simulink library "ProjectBlocks"  (R2016a)
settings: Solver=ode45  StartTime=0.0  StopTime=10.0  RelTol=1e-3
libraries: elec_lib x47, ProjectBlocks x9, SimscapeMacros x4, simulink x2, simulink_extras x1
settings Model: Creator=Peter  LastModifiedBy=Peter
settings DataIOCC: LimitDataPoints=on
settings DebuggingCC: AllowSymbolicDim=off

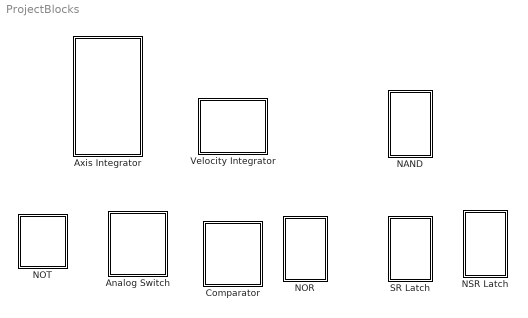
== system ProjectBlocks ==
  Analog Switch : Subsystem
  Axis Integrator : Subsystem
  Comparator : Subsystem
  NAND : Subsystem
  NOR : Subsystem
  NOT : Subsystem
  NSR Latch : Subsystem
  SR Latch : Subsystem
  Velocity Integrator : Subsystem

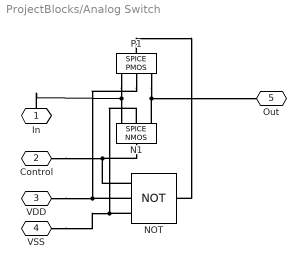
== system ProjectBlocks/Analog Switch ==
  N1 : elec_lib/Additional Components/SPICE-Compatible Components/Semiconductor Devices/SPICE NMOS  AREA=1  SCALE=1  LENGTH=7.8e-6 m  WIDTH=0.138e-3 m  AD=0.161e-8 m^2  AS=0.603e-8 m^2  PD=0 m  PS=0.478e-3 m  NRD=0.3  NRS=1  LEVEL=1  VTO=0.750 V  KP=NaN A/V^2  GAMMA=1.03 V^0.50000  PHI=0.70 V  LAMBDA=0.018 1/V  RD=NaN Ohm  RS=NaN Ohm  C_param=1  CBD=1e-18 F  CBS=1e-18 F  IS=1.206e-13 A  ND=1  PB=0.9 V  CGSO=0.94e-9 F/m  CGDO=0.59e-9 F/m  CGBO=0.138e-9 F/m  RSH=10 Ohm  CJ=0.39e-3 F/m^2  MJ=0.5  CJSW=264e-12 F/m  MJSW=0.18  JS=20e-6 A/m^2  TOX=0.055e-6 m  LD=1.6e-6 m  U0=650 cm^2/s/V  FC=0.5  NSUB=1e16 1/cm^3  TPG=1  NSS=0.7e11 1/cm^2  UEXP=0  UCRIT=1e+4 V/cm  NEFF=1  DELTA=0  VMAX=1.6e5 m/s  XJ=2.0e-6 m  NFS=1.17e11 1/cm^2  ETA=0  THETA=0 1/V  KAPPA=0.2  T_param=1  TOFFSET=0 K  TFIXED=300.15 K  TMEAS=300.15 K  IC_given=1  ICVDS=0 V  ICVGS=0 V  ICVBS=0 V  MTYPE=1
  NOT : ProjectBlocks/NOT
  P1 : elec_lib/Additional Components/SPICE-Compatible Components/Semiconductor Devices/SPICE PMOS  AREA=1  SCALE=1  LENGTH=7.8e-6 m  WIDTH=0.138e-3 m  AD=0.161e-8 m^2  AS=0.603e-8 m^2  PD=0 m  PS=0.478e-3 m  NRD=0.3  NRS=1  LEVEL=1  VTO=-0.74 V  KP=NaN A/V^2  GAMMA=0.58 V^0.50000  PHI=0.70 V  LAMBDA=.026 1/V  RD=NaN Ohm  RS=NaN Ohm  C_param=1  CBD=1e-18 F  CBS=1e-18 F  IS=1.206e-13 A  ND=1  PB=0.90 V  CGSO=0.31e-9 F/m  CGDO=0.39e-9 F/m  CGBO=0.138e-9 F/m  RSH=90 Ohm  CJ=0.18e-3 F/m^2  MJ=0.57  CJSW=322e-12 F/m  MJSW=0.33  JS=20e-6 A/m^2  TOX=0.055e-6 m  LD=0.96e-6 m  U0=260 cm^2/s/V  FC=0.5  NSUB=1e16 1/cm^3  TPG=-1  NSS=1e11 1/cm^2  UEXP=0  UCRIT=1e+4 V/cm  NEFF=1  DELTA=0  VMAX=3.0e5 m/s  XJ=1.2e-6 m  NFS=1.06e11 1/cm^2  ETA=0  THETA=0 1/V  KAPPA=0.2  T_param=1  TOFFSET=0 K  TFIXED=300.15 K  TMEAS=300.15 K  IC_given=1  ICVDS=0 V  ICVGS=0 V  ICVBS=0 V  MTYPE=-1
  In : PMIOPort  Port=1  Side=Left
  Control : PMIOPort  Port=2  Side=Left
  VDD : PMIOPort  Port=3  Side=Left
  VSS : PMIOPort  Port=4  Side=Left
  Out : PMIOPort  Port=5  Side=Right
  connections:
  P1/RConn1 -- In/RConn1 -- N1/RConn1
  N1/RConn3 -- Out/RConn1 -- P1/RConn3
  VDD/RConn1 -- NOT/LConn2 -- P1/RConn2
  VSS/RConn1 -- NOT/LConn3 -- N1/RConn2
  P1/LConn1 -- NOT/RConn1
  N1/LConn1 -- NOT/LConn1 -- Control/RConn1

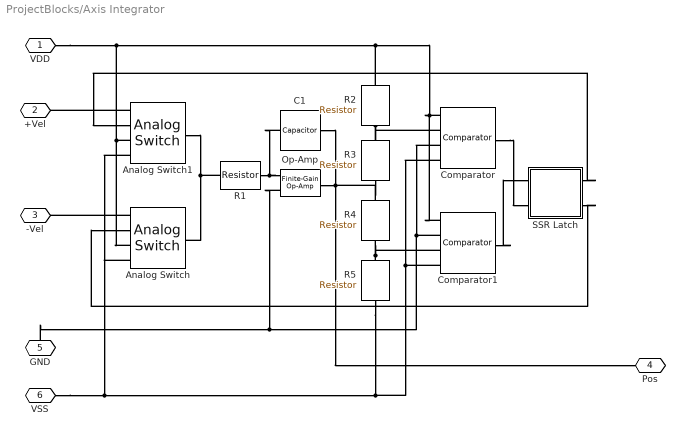
== system ProjectBlocks/Axis Integrator ==
  Analog Switch : ProjectBlocks/Analog Switch
  Analog Switch1 : ProjectBlocks/Analog Switch
  C1 : elec_lib/Passive Devices/Capacitor  enable_table=0  c=1e-6 F  Cvec=[ 1e-5 1e-6 ] F  Vvec=[ 0 10 ] V  CV_table_symmetry=1  C_tol=5  enable_C_tol=0  tol_distribution=1  nSigma=4  r=1e-6 Ohm  g=0 1/Ohm  initV=0 V  enable_operating_limits=0  operating_limit_action=2  max_working_voltage_range=[ -25 25 ] V  power_rating=1 W  enable_faults=0  fault_action=1  Cscale_faulted=100  R_faulted=0.001 Ohm  G_faulted=0 1/Ohm  tau_fault=0.001 s  enable_temporal_fault=0  t_fault=1 s  enable_behavioral_fault=0  max_permissible_voltage_range=[ -100 100 ] V  t_fail_on_voltage=1 s
  Comparator : ProjectBlocks/Comparator
  Comparator1 : ProjectBlocks/Comparator
  Op-Amp : elec_lib/Integrated Circuits/Finite-Gain Op-Amp  A=1000  Rin=1e6 Ohm  Rout=100 Ohm  Vmin=-10 V  Vmax=10 V
  R1 : elec_lib/Passive Devices/Resistor  R=100e3 Ohm  R_tol=5  enable_R_tol=0  tol_distribution=1  nSigma=4  enable_operating_limits=0  operating_limit_action=2  max_working_voltage=100 V  power_rating=1 W  enable_faults=0  fault_action=1  R_faulted=Inf Ohm  enable_temporal_fault=0  t_fault=1 s  enable_behavioral_fault=0  max_permissible_current=1 A  t_fail_on_current=1 s  noise_mode=0  sample_time=0.001 s  repeatability=1  auto_seed=736455394  user_seed=0  Tdevice=25 degC  alpha=0.00393 1/K  Tmeas=25 degC  thermal_mass=100 J/K  initial_temperature=25 degC  power_derating_T1=70 degC  power_derating_T2=155 degC  operating_temperature_range_vec=[ -50 150 ] degC
  R2 : elec_lib/Passive Devices/Resistor  R=10e3 Ohm  R_tol=5  enable_R_tol=0  tol_distribution=1  nSigma=4  enable_operating_limits=0  operating_limit_action=2  max_working_voltage=100 V  power_rating=1 W  enable_faults=0  fault_action=1  R_faulted=Inf Ohm  enable_temporal_fault=0  t_fault=1 s  enable_behavioral_fault=0  max_permissible_current=1 A  t_fail_on_current=1 s  noise_mode=0  sample_time=0.001 s  repeatability=1  auto_seed=38756620  user_seed=0  Tdevice=25 degC  alpha=0.00393 1/K  Tmeas=25 degC  thermal_mass=100 J/K  initial_temperature=25 degC  power_derating_T1=70 degC  power_derating_T2=155 degC  operating_temperature_range_vec=[ -50 150 ] degC
  R3 : elec_lib/Passive Devices/Resistor  R=5e3 Ohm  R_tol=5  enable_R_tol=0  tol_distribution=1  nSigma=4  enable_operating_limits=0  operating_limit_action=2  max_working_voltage=100 V  power_rating=1 W  enable_faults=0  fault_action=1  R_faulted=Inf Ohm  enable_temporal_fault=0  t_fault=1 s  enable_behavioral_fault=0  max_permissible_current=1 A  t_fail_on_current=1 s  noise_mode=0  sample_time=0.001 s  repeatability=1  auto_seed=726180734  user_seed=0  Tdevice=25 degC  alpha=0.00393 1/K  Tmeas=25 degC  thermal_mass=100 J/K  initial_temperature=25 degC  power_derating_T1=70 degC  power_derating_T2=155 degC  operating_temperature_range_vec=[ -50 150 ] degC
  R4 : elec_lib/Passive Devices/Resistor  R=5e3 Ohm  R_tol=5  enable_R_tol=0  tol_distribution=1  nSigma=4  enable_operating_limits=0  operating_limit_action=2  max_working_voltage=100 V  power_rating=1 W  enable_faults=0  fault_action=1  R_faulted=Inf Ohm  enable_temporal_fault=0  t_fault=1 s  enable_behavioral_fault=0  max_permissible_current=1 A  t_fail_on_current=1 s  noise_mode=0  sample_time=0.001 s  repeatability=1  auto_seed=886428727  user_seed=0  Tdevice=25 degC  alpha=0.00393 1/K  Tmeas=25 degC  thermal_mass=100 J/K  initial_temperature=25 degC  power_derating_T1=70 degC  power_derating_T2=155 degC  operating_temperature_range_vec=[ -50 150 ] degC
  R5 : elec_lib/Passive Devices/Resistor  R=10e3 Ohm  R_tol=5  enable_R_tol=0  tol_distribution=1  nSigma=4  enable_operating_limits=0  operating_limit_action=2  max_working_voltage=100 V  power_rating=1 W  enable_faults=0  fault_action=1  R_faulted=Inf Ohm  enable_temporal_fault=0  t_fault=1 s  enable_behavioral_fault=0  max_permissible_current=1 A  t_fail_on_current=1 s  noise_mode=0  sample_time=0.001 s  repeatability=1  auto_seed=3872437814  user_seed=0  Tdevice=25 degC  alpha=0.00393 1/K  Tmeas=25 degC  thermal_mass=100 J/K  initial_temperature=25 degC  power_derating_T1=70 degC  power_derating_T2=155 degC  operating_temperature_range_vec=[ -50 150 ] degC
  SSR Latch : Subsystem
  VDD : PMIOPort  Port=1  Side=Left
  +Vel : PMIOPort  Port=2  Side=Left
  -Vel : PMIOPort  Port=3  Side=Left
  Pos : PMIOPort  Port=4  Side=Right
  GND : PMIOPort  Port=5  Side=Left
  VSS : PMIOPort  Port=6  Side=Left
  connections:
  R1/RConn1 -- Op-Amp/LConn2 -- C1/RConn1
  Comparator/LConn4 -- Comparator1/LConn4 -- R5/RConn1 -- Analog Switch/LConn4 -- Analog Switch1/LConn4 -- VSS/RConn1
  Analog Switch/LConn3 -- Analog Switch1/LConn3 -- R2/LConn1 -- Comparator/LConn1 -- Comparator1/LConn1 -- VDD/RConn1
  R3/LConn1 -- R2/RConn1 -- Comparator/LConn2
  Op-Amp/LConn1 -- Comparator/LConn3 -- Comparator1/LConn2 -- GND/RConn1
  Analog Switch/LConn1 -- -Vel/RConn1
  Analog Switch1/LConn1 -- +Vel/RConn1
  R4/RConn1 -- R5/LConn1 -- Comparator1/LConn3
  R1/LConn1 -- Analog Switch1/RConn1 -- Analog Switch/RConn1
  C1/LConn1 -- R3/RConn1 -- R4/LConn1 -- Op-Amp/RConn1 -- Pos/RConn1
  SSR Latch/RConn2 -- Analog Switch/LConn2
  SSR Latch/RConn1 -- Analog Switch1/LConn2
  Comparator/RConn1 -- SSR Latch/LConn2
  Comparator1/RConn1 -- SSR Latch/LConn1

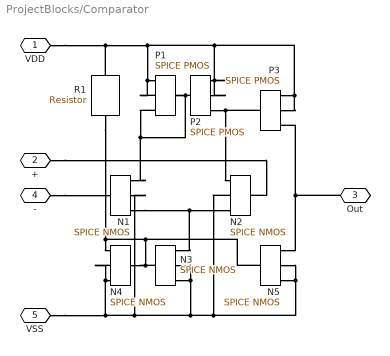
== system ProjectBlocks/Comparator ==
  N{1..5} (5 alike) : elec_lib/Additional Components/SPICE-Compatible Components/Semiconductor Devices/SPICE NMOS  AREA=1  SCALE=1  LENGTH=7.8e-6 m  WIDTH=0.138e-3 m  AD=0.161e-8 m^2  AS=0.603e-8 m^2  PD=0 m  PS=0.478e-3 m  NRD=0.3  NRS=1  LEVEL=1  VTO=0.750 V  KP=NaN A/V^2  GAMMA=1.03 V^0.50000  PHI=0.70 V  LAMBDA=0.018 1/V  RD=NaN Ohm  RS=NaN Ohm  C_param=1  CBD=1e-18 F  CBS=1e-18 F  IS=1.206e-13 A  ND=1  PB=0.9 V  CGSO=0.94e-9 F/m  CGDO=0.59e-9 F/m  CGBO=0.138e-9 F/m  RSH=10 Ohm  CJ=0.39e-3 F/m^2  MJ=0.5  CJSW=264e-12 F/m  MJSW=0.18  JS=20e-6 A/m^2  TOX=0.055e-6 m  LD=1.6e-6 m  U0=650 cm^2/s/V  FC=0.5  NSUB=1e16 1/cm^3  TPG=1  NSS=0.7e11 1/cm^2  UEXP=0  UCRIT=1e+4 V/cm  NEFF=1  DELTA=0  VMAX=1.6e5 m/s  XJ=2.0e-6 m  NFS=1.17e11 1/cm^2  ETA=0  THETA=0 1/V  KAPPA=0.2  T_param=1  TOFFSET=0 K  TFIXED=300.15 K  TMEAS=300.15 K  IC_given=1  ICVDS=0 V  ICVGS=0 V  ICVBS=0 V  MTYPE=1
  P1 : elec_lib/Additional Components/SPICE-Compatible Components/Semiconductor Devices/SPICE PMOS  AREA=1  SCALE=1  LENGTH=7.8e-6 m  WIDTH=0.138e-3 m  AD=0.161e-8 m^2  AS=0.603e-8 m^2  PD=0 m  PS=0.478e-3 m  NRD=0.3  NRS=1  LEVEL=1  VTO=-0.74 V  KP=NaN A/V^2  GAMMA=0.58 V^0.50000  PHI=0.70 V  LAMBDA=.026 1/V  RD=NaN Ohm  RS=NaN Ohm  C_param=1  CBD=1e-18 F  CBS=1e-18 F  IS=1.206e-13 A  ND=1  PB=0.90 V  CGSO=0.31e-9 F/m  CGDO=0.39e-9 F/m  CGBO=0.138e-9 F/m  RSH=90 Ohm  CJ=0.18e-3 F/m^2  MJ=0.57  CJSW=322e-12 F/m  MJSW=0.33  JS=20e-6 A/m^2  TOX=0.055e-6 m  LD=0.96e-6 m  U0=260 cm^2/s/V  FC=0.5  NSUB=1e16 1/cm^3  TPG=-1  NSS=1e11 1/cm^2  UEXP=0  UCRIT=1e+4 V/cm  NEFF=1  DELTA=0  VMAX=3.0e5 m/s  XJ=1.2e-6 m  NFS=1.06e11 1/cm^2  ETA=0  THETA=0 1/V  KAPPA=0.2  T_param=1  TOFFSET=0 K  TFIXED=300.15 K  TMEAS=300.15 K  IC_given=1  ICVDS=0 V  ICVGS=0 V  ICVBS=0 V  MTYPE=-1
  P2 : elec_lib/Additional Components/SPICE-Compatible Components/Semiconductor Devices/SPICE PMOS  AREA=1  SCALE=1  LENGTH=7.8e-6 m  WIDTH=0.138e-3 m  AD=0.161e-8 m^2  AS=0.603e-8 m^2  PD=0 m  PS=0.478e-3 m  NRD=0.3  NRS=1  LEVEL=1  VTO=-0.74 V  KP=NaN A/V^2  GAMMA=0.58 V^0.50000  PHI=0.70 V  LAMBDA=.026 1/V  RD=NaN Ohm  RS=NaN Ohm  C_param=1  CBD=1e-18 F  CBS=1e-18 F  IS=1.206e-13 A  ND=1  PB=0.90 V  CGSO=0.31e-9 F/m  CGDO=0.39e-9 F/m  CGBO=0.138e-9 F/m  RSH=90 Ohm  CJ=0.18e-3 F/m^2  MJ=0.57  CJSW=322e-12 F/m  MJSW=0.33  JS=20e-6 A/m^2  TOX=0.055e-6 m  LD=0.96e-6 m  U0=260 cm^2/s/V  FC=0.5  NSUB=1e16 1/cm^3  TPG=-1  NSS=1e11 1/cm^2  UEXP=0  UCRIT=1e+4 V/cm  NEFF=1  DELTA=0  VMAX=3.0e5 m/s  XJ=1.2e-6 m  NFS=1.06e11 1/cm^2  ETA=0  THETA=0 1/V  KAPPA=0.2  T_param=1  TOFFSET=0 K  TFIXED=300.15 K  TMEAS=300.15 K  IC_given=1  ICVDS=0 V  ICVGS=0 V  ICVBS=0 V  MTYPE=-1
  P3 : elec_lib/Additional Components/SPICE-Compatible Components/Semiconductor Devices/SPICE PMOS  AREA=1  SCALE=1  LENGTH=7.8e-6 m  WIDTH=0.138e-3 m  AD=0.161e-8 m^2  AS=0.603e-8 m^2  PD=0 m  PS=0.478e-3 m  NRD=0.3  NRS=1  LEVEL=1  VTO=-0.74 V  KP=NaN A/V^2  GAMMA=0.58 V^0.50000  PHI=0.70 V  LAMBDA=.026 1/V  RD=NaN Ohm  RS=NaN Ohm  C_param=1  CBD=1e-18 F  CBS=1e-18 F  IS=1.206e-13 A  ND=1  PB=0.90 V  CGSO=0.31e-9 F/m  CGDO=0.39e-9 F/m  CGBO=0.138e-9 F/m  RSH=90 Ohm  CJ=0.18e-3 F/m^2  MJ=0.57  CJSW=322e-12 F/m  MJSW=0.33  JS=20e-6 A/m^2  TOX=0.055e-6 m  LD=0.96e-6 m  U0=260 cm^2/s/V  FC=0.5  NSUB=1e16 1/cm^3  TPG=-1  NSS=1e11 1/cm^2  UEXP=0  UCRIT=1e+4 V/cm  NEFF=1  DELTA=0  VMAX=3.0e5 m/s  XJ=1.2e-6 m  NFS=1.06e11 1/cm^2  ETA=0  THETA=0 1/V  KAPPA=0.2  T_param=1  TOFFSET=0 K  TFIXED=300.15 K  TMEAS=300.15 K  IC_given=1  ICVDS=0 V  ICVGS=0 V  ICVBS=0 V  MTYPE=-1
  R1 : elec_lib/Passive Devices/Resistor  R=72e3 Ohm  R_tol=5  enable_R_tol=0  tol_distribution=1  nSigma=4  enable_operating_limits=0  operating_limit_action=2  max_working_voltage=100 V  power_rating=1 W  enable_faults=0  fault_action=1  R_faulted=Inf Ohm  enable_temporal_fault=0  t_fault=1 s  enable_behavioral_fault=0  max_permissible_current=1 A  t_fail_on_current=1 s  noise_mode=0  sample_time=0.001 s  repeatability=1  auto_seed=1225241502  user_seed=0  Tdevice=25 degC  alpha=0.00393 1/K  Tmeas=25 degC  thermal_mass=100 J/K  initial_temperature=25 degC  power_derating_T1=70 degC  power_derating_T2=155 degC  operating_temperature_range_vec=[ -50 150 ] degC
  VDD : PMIOPort  Port=1  Side=Left
  + : PMIOPort  Port=2  Side=Left
  Out : PMIOPort  Port=3  Side=Right
  - : PMIOPort  Port=4  Side=Left
  VSS : PMIOPort  Port=5  Side=Left
  connections:
  VSS/RConn1 -- N2/RConn2 -- N5/RConn2 -- N5/RConn1 -- N3/RConn2 -- N3/RConn1 -- N1/RConn2 -- N4/RConn2 -- N4/RConn1
  R1/RConn1 -- N3/LConn1 -- N4/LConn1 -- N5/LConn1 -- N4/RConn3
  N5/RConn3 -- Out/RConn1 -- P3/RConn3
  P2/RConn3 -- P3/LConn1 -- N2/RConn3
  +/RConn1 -- N2/LConn1
  -/RConn1 -- N1/LConn1
  P1/RConn3 -- N1/RConn3 -- P2/LConn1 -- P1/LConn1
  P2/RConn1 -- P3/RConn2 -- P3/RConn1 -- VDD/RConn1 -- R1/LConn1 -- P1/RConn2 -- P1/RConn1 -- P2/RConn2
  N1/RConn1 -- N3/RConn3 -- N2/RConn1

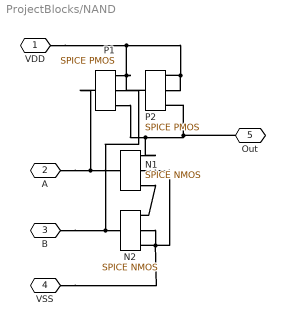
== system ProjectBlocks/NAND ==
  N1 : elec_lib/Additional Components/SPICE-Compatible Components/Semiconductor Devices/SPICE NMOS  AREA=1  SCALE=1  LENGTH=7.8e-6 m  WIDTH=0.138e-3 m  AD=0.161e-8 m^2  AS=0.603e-8 m^2  PD=0 m  PS=0.478e-3 m  NRD=0.3  NRS=1  LEVEL=1  VTO=0.750 V  KP=NaN A/V^2  GAMMA=1.03 V^0.50000  PHI=0.70 V  LAMBDA=0.018 1/V  RD=NaN Ohm  RS=NaN Ohm  C_param=1  CBD=1e-18 F  CBS=1e-18 F  IS=1.206e-13 A  ND=1  PB=0.9 V  CGSO=0.94e-9 F/m  CGDO=0.59e-9 F/m  CGBO=0.138e-9 F/m  RSH=10 Ohm  CJ=0.39e-3 F/m^2  MJ=0.5  CJSW=264e-12 F/m  MJSW=0.18  JS=20e-6 A/m^2  TOX=0.055e-6 m  LD=1.6e-6 m  U0=650 cm^2/s/V  FC=0.5  NSUB=1e16 1/cm^3  TPG=1  NSS=0.7e11 1/cm^2  UEXP=0  UCRIT=1e+4 V/cm  NEFF=1  DELTA=0  VMAX=1.6e5 m/s  XJ=2.0e-6 m  NFS=1.17e11 1/cm^2  ETA=0  THETA=0 1/V  KAPPA=0.2  T_param=1  TOFFSET=0 K  TFIXED=300.15 K  TMEAS=300.15 K  IC_given=1  ICVDS=0 V  ICVGS=0 V  ICVBS=0 V  MTYPE=1
  N2 : elec_lib/Additional Components/SPICE-Compatible Components/Semiconductor Devices/SPICE NMOS  AREA=1  SCALE=1  LENGTH=7.8e-6 m  WIDTH=0.138e-3 m  AD=0.161e-8 m^2  AS=0.603e-8 m^2  PD=0 m  PS=0.478e-3 m  NRD=0.3  NRS=1  LEVEL=1  VTO=0.750 V  KP=NaN A/V^2  GAMMA=1.03 V^0.50000  PHI=0.70 V  LAMBDA=0.018 1/V  RD=NaN Ohm  RS=NaN Ohm  C_param=1  CBD=1e-18 F  CBS=1e-18 F  IS=1.206e-13 A  ND=1  PB=0.9 V  CGSO=0.94e-9 F/m  CGDO=0.59e-9 F/m  CGBO=0.138e-9 F/m  RSH=10 Ohm  CJ=0.39e-3 F/m^2  MJ=0.5  CJSW=264e-12 F/m  MJSW=0.18  JS=20e-6 A/m^2  TOX=0.055e-6 m  LD=1.6e-6 m  U0=650 cm^2/s/V  FC=0.5  NSUB=1e16 1/cm^3  TPG=1  NSS=0.7e11 1/cm^2  UEXP=0  UCRIT=1e+4 V/cm  NEFF=1  DELTA=0  VMAX=1.6e5 m/s  XJ=2.0e-6 m  NFS=1.17e11 1/cm^2  ETA=0  THETA=0 1/V  KAPPA=0.2  T_param=1  TOFFSET=0 K  TFIXED=300.15 K  TMEAS=300.15 K  IC_given=1  ICVDS=0 V  ICVGS=0 V  ICVBS=0 V  MTYPE=1
  P1 : elec_lib/Additional Components/SPICE-Compatible Components/Semiconductor Devices/SPICE PMOS  AREA=1  SCALE=1  LENGTH=7.8e-6 m  WIDTH=0.138e-3 m  AD=0.161e-8 m^2  AS=0.603e-8 m^2  PD=0 m  PS=0.478e-3 m  NRD=0.3  NRS=1  LEVEL=1  VTO=-0.74 V  KP=NaN A/V^2  GAMMA=0.58 V^0.50000  PHI=0.70 V  LAMBDA=.026 1/V  RD=NaN Ohm  RS=NaN Ohm  C_param=1  CBD=1e-18 F  CBS=1e-18 F  IS=1.206e-13 A  ND=1  PB=0.90 V  CGSO=0.31e-9 F/m  CGDO=0.39e-9 F/m  CGBO=0.138e-9 F/m  RSH=90 Ohm  CJ=0.18e-3 F/m^2  MJ=0.57  CJSW=322e-12 F/m  MJSW=0.33  JS=20e-6 A/m^2  TOX=0.055e-6 m  LD=0.96e-6 m  U0=260 cm^2/s/V  FC=0.5  NSUB=1e16 1/cm^3  TPG=-1  NSS=1e11 1/cm^2  UEXP=0  UCRIT=1e+4 V/cm  NEFF=1  DELTA=0  VMAX=3.0e5 m/s  XJ=1.2e-6 m  NFS=1.06e11 1/cm^2  ETA=0  THETA=0 1/V  KAPPA=0.2  T_param=1  TOFFSET=0 K  TFIXED=300.15 K  TMEAS=300.15 K  IC_given=1  ICVDS=0 V  ICVGS=0 V  ICVBS=0 V  MTYPE=-1
  P2 : elec_lib/Additional Components/SPICE-Compatible Components/Semiconductor Devices/SPICE PMOS  AREA=1  SCALE=1  LENGTH=7.8e-6 m  WIDTH=0.138e-3 m  AD=0.161e-8 m^2  AS=0.603e-8 m^2  PD=0 m  PS=0.478e-3 m  NRD=0.3  NRS=1  LEVEL=1  VTO=-0.74 V  KP=NaN A/V^2  GAMMA=0.58 V^0.50000  PHI=0.70 V  LAMBDA=.026 1/V  RD=NaN Ohm  RS=NaN Ohm  C_param=1  CBD=1e-18 F  CBS=1e-18 F  IS=1.206e-13 A  ND=1  PB=0.90 V  CGSO=0.31e-9 F/m  CGDO=0.39e-9 F/m  CGBO=0.138e-9 F/m  RSH=90 Ohm  CJ=0.18e-3 F/m^2  MJ=0.57  CJSW=322e-12 F/m  MJSW=0.33  JS=20e-6 A/m^2  TOX=0.055e-6 m  LD=0.96e-6 m  U0=260 cm^2/s/V  FC=0.5  NSUB=1e16 1/cm^3  TPG=-1  NSS=1e11 1/cm^2  UEXP=0  UCRIT=1e+4 V/cm  NEFF=1  DELTA=0  VMAX=3.0e5 m/s  XJ=1.2e-6 m  NFS=1.06e11 1/cm^2  ETA=0  THETA=0 1/V  KAPPA=0.2  T_param=1  TOFFSET=0 K  TFIXED=300.15 K  TMEAS=300.15 K  IC_given=1  ICVDS=0 V  ICVGS=0 V  ICVBS=0 V  MTYPE=-1
  VDD : PMIOPort  Port=1  Side=Left
  A : PMIOPort  Port=2  Side=Left
  B : PMIOPort  Port=3  Side=Left
  VSS : PMIOPort  Port=4  Side=Left
  Out : PMIOPort  Port=5  Side=Right
  connections:
  VDD/RConn1 -- P1/RConn2 -- P1/RConn1 -- P2/RConn2 -- P2/RConn1
  N2/LConn1 -- B/RConn1 -- P2/LConn1
  N1/RConn1 -- N2/RConn3
  N2/RConn1 -- VSS/RConn1 -- N1/RConn2 -- N2/RConn2
  P1/RConn3 -- N1/RConn3 -- Out/RConn1 -- P2/RConn3
  N1/LConn1 -- A/RConn1 -- P1/LConn1

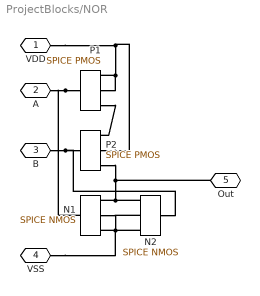
== system ProjectBlocks/NOR ==
  N1 : elec_lib/Additional Components/SPICE-Compatible Components/Semiconductor Devices/SPICE NMOS  AREA=1  SCALE=1  LENGTH=7.8e-6 m  WIDTH=0.138e-3 m  AD=0.161e-8 m^2  AS=0.603e-8 m^2  PD=0 m  PS=0.478e-3 m  NRD=0.3  NRS=1  LEVEL=1  VTO=0.750 V  KP=NaN A/V^2  GAMMA=1.03 V^0.50000  PHI=0.70 V  LAMBDA=0.018 1/V  RD=NaN Ohm  RS=NaN Ohm  C_param=1  CBD=1e-18 F  CBS=1e-18 F  IS=1.206e-13 A  ND=1  PB=0.9 V  CGSO=0.94e-9 F/m  CGDO=0.59e-9 F/m  CGBO=0.138e-9 F/m  RSH=10 Ohm  CJ=0.39e-3 F/m^2  MJ=0.5  CJSW=264e-12 F/m  MJSW=0.18  JS=20e-6 A/m^2  TOX=0.055e-6 m  LD=1.6e-6 m  U0=650 cm^2/s/V  FC=0.5  NSUB=1e16 1/cm^3  TPG=1  NSS=0.7e11 1/cm^2  UEXP=0  UCRIT=1e+4 V/cm  NEFF=1  DELTA=0  VMAX=1.6e5 m/s  XJ=2.0e-6 m  NFS=1.17e11 1/cm^2  ETA=0  THETA=0 1/V  KAPPA=0.2  T_param=1  TOFFSET=0 K  TFIXED=300.15 K  TMEAS=300.15 K  IC_given=1  ICVDS=0 V  ICVGS=0 V  ICVBS=0 V  MTYPE=1
  N2 : elec_lib/Additional Components/SPICE-Compatible Components/Semiconductor Devices/SPICE NMOS  AREA=1  SCALE=1  LENGTH=7.8e-6 m  WIDTH=0.138e-3 m  AD=0.161e-8 m^2  AS=0.603e-8 m^2  PD=0 m  PS=0.478e-3 m  NRD=0.3  NRS=1  LEVEL=1  VTO=0.750 V  KP=NaN A/V^2  GAMMA=1.03 V^0.50000  PHI=0.70 V  LAMBDA=0.018 1/V  RD=NaN Ohm  RS=NaN Ohm  C_param=1  CBD=1e-18 F  CBS=1e-18 F  IS=1.206e-13 A  ND=1  PB=0.9 V  CGSO=0.94e-9 F/m  CGDO=0.59e-9 F/m  CGBO=0.138e-9 F/m  RSH=10 Ohm  CJ=0.39e-3 F/m^2  MJ=0.5  CJSW=264e-12 F/m  MJSW=0.18  JS=20e-6 A/m^2  TOX=0.055e-6 m  LD=1.6e-6 m  U0=650 cm^2/s/V  FC=0.5  NSUB=1e16 1/cm^3  TPG=1  NSS=0.7e11 1/cm^2  UEXP=0  UCRIT=1e+4 V/cm  NEFF=1  DELTA=0  VMAX=1.6e5 m/s  XJ=2.0e-6 m  NFS=1.17e11 1/cm^2  ETA=0  THETA=0 1/V  KAPPA=0.2  T_param=1  TOFFSET=0 K  TFIXED=300.15 K  TMEAS=300.15 K  IC_given=1  ICVDS=0 V  ICVGS=0 V  ICVBS=0 V  MTYPE=1
  P1 : elec_lib/Additional Components/SPICE-Compatible Components/Semiconductor Devices/SPICE PMOS  AREA=1  SCALE=1  LENGTH=7.8e-6 m  WIDTH=0.138e-3 m  AD=0.161e-8 m^2  AS=0.603e-8 m^2  PD=0 m  PS=0.478e-3 m  NRD=0.3  NRS=1  LEVEL=1  VTO=-0.74 V  KP=NaN A/V^2  GAMMA=0.58 V^0.50000  PHI=0.70 V  LAMBDA=.026 1/V  RD=NaN Ohm  RS=NaN Ohm  C_param=1  CBD=1e-18 F  CBS=1e-18 F  IS=1.206e-13 A  ND=1  PB=0.90 V  CGSO=0.31e-9 F/m  CGDO=0.39e-9 F/m  CGBO=0.138e-9 F/m  RSH=90 Ohm  CJ=0.18e-3 F/m^2  MJ=0.57  CJSW=322e-12 F/m  MJSW=0.33  JS=20e-6 A/m^2  TOX=0.055e-6 m  LD=0.96e-6 m  U0=260 cm^2/s/V  FC=0.5  NSUB=1e16 1/cm^3  TPG=-1  NSS=1e11 1/cm^2  UEXP=0  UCRIT=1e+4 V/cm  NEFF=1  DELTA=0  VMAX=3.0e5 m/s  XJ=1.2e-6 m  NFS=1.06e11 1/cm^2  ETA=0  THETA=0 1/V  KAPPA=0.2  T_param=1  TOFFSET=0 K  TFIXED=300.15 K  TMEAS=300.15 K  IC_given=1  ICVDS=0 V  ICVGS=0 V  ICVBS=0 V  MTYPE=-1
  P2 : elec_lib/Additional Components/SPICE-Compatible Components/Semiconductor Devices/SPICE PMOS  AREA=1  SCALE=1  LENGTH=7.8e-6 m  WIDTH=0.138e-3 m  AD=0.161e-8 m^2  AS=0.603e-8 m^2  PD=0 m  PS=0.478e-3 m  NRD=0.3  NRS=1  LEVEL=1  VTO=-0.74 V  KP=NaN A/V^2  GAMMA=0.58 V^0.50000  PHI=0.70 V  LAMBDA=.026 1/V  RD=NaN Ohm  RS=NaN Ohm  C_param=1  CBD=1e-18 F  CBS=1e-18 F  IS=1.206e-13 A  ND=1  PB=0.90 V  CGSO=0.31e-9 F/m  CGDO=0.39e-9 F/m  CGBO=0.138e-9 F/m  RSH=90 Ohm  CJ=0.18e-3 F/m^2  MJ=0.57  CJSW=322e-12 F/m  MJSW=0.33  JS=20e-6 A/m^2  TOX=0.055e-6 m  LD=0.96e-6 m  U0=260 cm^2/s/V  FC=0.5  NSUB=1e16 1/cm^3  TPG=-1  NSS=1e11 1/cm^2  UEXP=0  UCRIT=1e+4 V/cm  NEFF=1  DELTA=0  VMAX=3.0e5 m/s  XJ=1.2e-6 m  NFS=1.06e11 1/cm^2  ETA=0  THETA=0 1/V  KAPPA=0.2  T_param=1  TOFFSET=0 K  TFIXED=300.15 K  TMEAS=300.15 K  IC_given=1  ICVDS=0 V  ICVGS=0 V  ICVBS=0 V  MTYPE=-1
  VDD : PMIOPort  Port=1  Side=Left
  A : PMIOPort  Port=2  Side=Left
  B : PMIOPort  Port=3  Side=Left
  VSS : PMIOPort  Port=4  Side=Left
  Out : PMIOPort  Port=5  Side=Right
  connections:
  P1/RConn3 -- P2/RConn1
  P2/RConn3 -- Out/RConn1 -- N2/RConn3 -- N1/RConn3
  B/RConn1 -- N2/LConn1 -- P2/LConn1
  A/RConn1 -- N1/LConn1 -- P1/LConn1
  VDD/RConn1 -- P2/RConn2 -- P1/RConn2 -- P1/RConn1
  VSS/RConn1 -- N2/RConn2 -- N1/RConn2 -- N2/RConn1 -- N1/RConn1

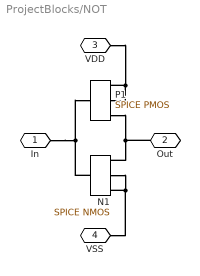
== system ProjectBlocks/NOT ==
  N1 : elec_lib/Additional Components/SPICE-Compatible Components/Semiconductor Devices/SPICE NMOS  AREA=1  SCALE=1  LENGTH=7.8e-6 m  WIDTH=0.138e-3 m  AD=0.161e-8 m^2  AS=0.603e-8 m^2  PD=0 m  PS=0.478e-3 m  NRD=0.3  NRS=1  LEVEL=1  VTO=0.750 V  KP=NaN A/V^2  GAMMA=1.03 V^0.50000  PHI=0.70 V  LAMBDA=0.018 1/V  RD=NaN Ohm  RS=NaN Ohm  C_param=1  CBD=1e-18 F  CBS=1e-18 F  IS=1.206e-13 A  ND=1  PB=0.9 V  CGSO=0.94e-9 F/m  CGDO=0.59e-9 F/m  CGBO=0.138e-9 F/m  RSH=10 Ohm  CJ=0.39e-3 F/m^2  MJ=0.5  CJSW=264e-12 F/m  MJSW=0.18  JS=20e-6 A/m^2  TOX=0.055e-6 m  LD=1.6e-6 m  U0=650 cm^2/s/V  FC=0.5  NSUB=1e16 1/cm^3  TPG=1  NSS=0.7e11 1/cm^2  UEXP=0  UCRIT=1e+4 V/cm  NEFF=1  DELTA=0  VMAX=1.6e5 m/s  XJ=2.0e-6 m  NFS=1.17e11 1/cm^2  ETA=0  THETA=0 1/V  KAPPA=0.2  T_param=1  TOFFSET=0 K  TFIXED=300.15 K  TMEAS=300.15 K  IC_given=1  ICVDS=0 V  ICVGS=0 V  ICVBS=0 V  MTYPE=1
  P1 : elec_lib/Additional Components/SPICE-Compatible Components/Semiconductor Devices/SPICE PMOS  AREA=1  SCALE=1  LENGTH=7.8e-6 m  WIDTH=0.138e-3 m  AD=0.161e-8 m^2  AS=0.603e-8 m^2  PD=0 m  PS=0.478e-3 m  NRD=0.3  NRS=1  LEVEL=1  VTO=-0.74 V  KP=NaN A/V^2  GAMMA=0.58 V^0.50000  PHI=0.70 V  LAMBDA=.026 1/V  RD=NaN Ohm  RS=NaN Ohm  C_param=1  CBD=1e-18 F  CBS=1e-18 F  IS=1.206e-13 A  ND=1  PB=0.90 V  CGSO=0.31e-9 F/m  CGDO=0.39e-9 F/m  CGBO=0.138e-9 F/m  RSH=90 Ohm  CJ=0.18e-3 F/m^2  MJ=0.57  CJSW=322e-12 F/m  MJSW=0.33  JS=20e-6 A/m^2  TOX=0.055e-6 m  LD=0.96e-6 m  U0=260 cm^2/s/V  FC=0.5  NSUB=1e16 1/cm^3  TPG=-1  NSS=1e11 1/cm^2  UEXP=0  UCRIT=1e+4 V/cm  NEFF=1  DELTA=0  VMAX=3.0e5 m/s  XJ=1.2e-6 m  NFS=1.06e11 1/cm^2  ETA=0  THETA=0 1/V  KAPPA=0.2  T_param=1  TOFFSET=0 K  TFIXED=300.15 K  TMEAS=300.15 K  IC_given=1  ICVDS=0 V  ICVGS=0 V  ICVBS=0 V  MTYPE=-1
  In : PMIOPort  Port=1  Side=Left
  Out : PMIOPort  Port=2  Side=Right
  VDD : PMIOPort  Port=3  Side=Left
  VSS : PMIOPort  Port=4  Side=Left
  connections:
  P1/RConn3 -- Out/RConn1 -- N1/RConn3
  N1/LConn1 -- In/RConn1 -- P1/LConn1
  P1/RConn2 -- VDD/RConn1 -- P1/RConn1
  N1/RConn2 -- VSS/RConn1 -- N1/RConn1

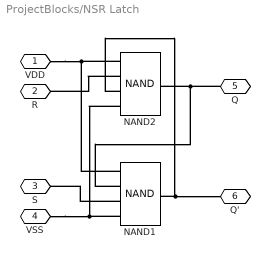
== system ProjectBlocks/NSR Latch ==
  NAND1 : ProjectBlocks/NAND
  NAND2 : ProjectBlocks/NAND
  VDD : PMIOPort  Port=1  Side=Left
  R : PMIOPort  Port=2  Side=Left
  S : PMIOPort  Port=3  Side=Left
  VSS : PMIOPort  Port=4  Side=Left
  Q : PMIOPort  Port=5  Side=Right
  Q' : PMIOPort  Port=6  Side=Right
  connections:
  NAND1/LConn1 -- VDD/RConn1 -- NAND2/LConn1
  NAND1/LConn3 -- S/RConn1
  NAND2/LConn2 -- R/RConn1
  NAND1/LConn2 -- Q/RConn1 -- NAND2/RConn1
  NAND1/RConn1 -- Q'/RConn1 -- NAND2/LConn3
  NAND1/LConn4 -- VSS/RConn1 -- NAND2/LConn4

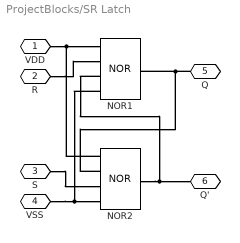
== system ProjectBlocks/SR Latch ==
  NOR1 : ProjectBlocks/NOR
  NOR2 : ProjectBlocks/NOR
  VDD : PMIOPort  Port=1  Side=Left
  R : PMIOPort  Port=2  Side=Left
  S : PMIOPort  Port=3  Side=Left
  VSS : PMIOPort  Port=4  Side=Left
  Q : PMIOPort  Port=5  Side=Right
  Q' : PMIOPort  Port=6  Side=Right
  connections:
  NOR2/RConn1 -- Q'/RConn1 -- NOR1/LConn3
  Q/RConn1 -- NOR1/RConn1 -- NOR2/LConn2
  VSS/RConn1 -- NOR1/LConn4 -- NOR2/LConn4
  VDD/RConn1 -- NOR2/LConn1 -- NOR1/LConn1
  R/RConn1 -- NOR1/LConn2
  S/RConn1 -- NOR2/LConn3

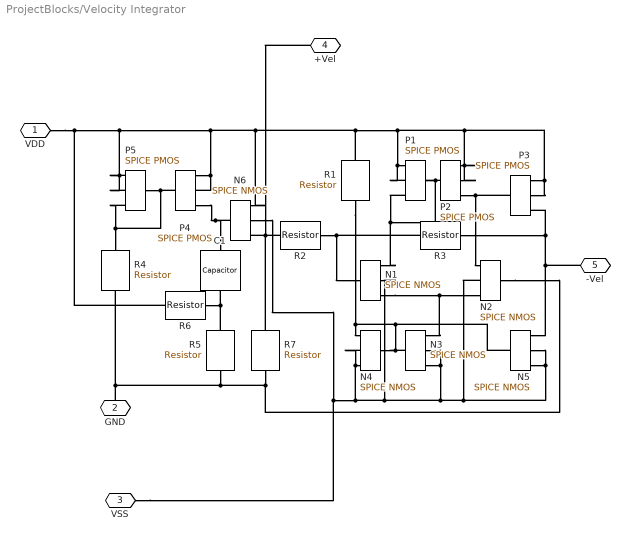
== system ProjectBlocks/Velocity Integrator ==
  C1 : elec_lib/Passive Devices/Capacitor  enable_table=0  c=220e-6 F  Cvec=[ 1e-5 1e-6 ] F  Vvec=[ 0 10 ] V  CV_table_symmetry=1  C_tol=5  enable_C_tol=0  tol_distribution=1  nSigma=4  r=1e-6 Ohm  g=0 1/Ohm  initV=0 V  enable_operating_limits=0  operating_limit_action=2  max_working_voltage_range=[ -25 25 ] V  power_rating=1 W  enable_faults=0  fault_action=1  Cscale_faulted=100  R_faulted=0.001 Ohm  G_faulted=0 1/Ohm  tau_fault=0.001 s  enable_temporal_fault=0  t_fault=1 s  enable_behavioral_fault=0  max_permissible_voltage_range=[ -100 100 ] V  t_fail_on_voltage=1 s
  N{1..6} (6 alike) : elec_lib/Additional Components/SPICE-Compatible Components/Semiconductor Devices/SPICE NMOS  AREA=1  SCALE=1  LENGTH=7.8e-6 m  WIDTH=0.138e-3 m  AD=0.161e-8 m^2  AS=0.603e-8 m^2  PD=0 m  PS=0.478e-3 m  NRD=0.3  NRS=1  LEVEL=1  VTO=0.750 V  KP=NaN A/V^2  GAMMA=1.03 V^0.50000  PHI=0.70 V  LAMBDA=0.018 1/V  RD=NaN Ohm  RS=NaN Ohm  C_param=1  CBD=1e-18 F  CBS=1e-18 F  IS=1.206e-13 A  ND=1  PB=0.9 V  CGSO=0.94e-9 F/m  CGDO=0.59e-9 F/m  CGBO=0.138e-9 F/m  RSH=10 Ohm  CJ=0.39e-3 F/m^2  MJ=0.5  CJSW=264e-12 F/m  MJSW=0.18  JS=20e-6 A/m^2  TOX=0.055e-6 m  LD=1.6e-6 m  U0=650 cm^2/s/V  FC=0.5  NSUB=1e16 1/cm^3  TPG=1  NSS=0.7e11 1/cm^2  UEXP=0  UCRIT=1e+4 V/cm  NEFF=1  DELTA=0  VMAX=1.6e5 m/s  XJ=2.0e-6 m  NFS=1.17e11 1/cm^2  ETA=0  THETA=0 1/V  KAPPA=0.2  T_param=1  TOFFSET=0 K  TFIXED=300.15 K  TMEAS=300.15 K  IC_given=1  ICVDS=0 V  ICVGS=0 V  ICVBS=0 V  MTYPE=1
  P{1..5} (5 alike) : elec_lib/Additional Components/SPICE-Compatible Components/Semiconductor Devices/SPICE PMOS  AREA=1  SCALE=1  LENGTH=7.8e-6 m  WIDTH=0.138e-3 m  AD=0.161e-8 m^2  AS=0.603e-8 m^2  PD=0 m  PS=0.478e-3 m  NRD=0.3  NRS=1  LEVEL=1  VTO=-0.74 V  KP=NaN A/V^2  GAMMA=0.58 V^0.50000  PHI=0.70 V  LAMBDA=.026 1/V  RD=NaN Ohm  RS=NaN Ohm  C_param=1  CBD=1e-18 F  CBS=1e-18 F  IS=1.206e-13 A  ND=1  PB=0.90 V  CGSO=0.31e-9 F/m  CGDO=0.39e-9 F/m  CGBO=0.138e-9 F/m  RSH=90 Ohm  CJ=0.18e-3 F/m^2  MJ=0.57  CJSW=322e-12 F/m  MJSW=0.33  JS=20e-6 A/m^2  TOX=0.055e-6 m  LD=0.96e-6 m  U0=260 cm^2/s/V  FC=0.5  NSUB=1e16 1/cm^3  TPG=-1  NSS=1e11 1/cm^2  UEXP=0  UCRIT=1e+4 V/cm  NEFF=1  DELTA=0  VMAX=3.0e5 m/s  XJ=1.2e-6 m  NFS=1.06e11 1/cm^2  ETA=0  THETA=0 1/V  KAPPA=0.2  T_param=1  TOFFSET=0 K  TFIXED=300.15 K  TMEAS=300.15 K  IC_given=1  ICVDS=0 V  ICVGS=0 V  ICVBS=0 V  MTYPE=-1
  R1 : elec_lib/Passive Devices/Resistor  R=72e3 Ohm  R_tol=5  enable_R_tol=0  tol_distribution=1  nSigma=4  enable_operating_limits=0  operating_limit_action=2  max_working_voltage=100 V  power_rating=1 W  enable_faults=0  fault_action=1  R_faulted=Inf Ohm  enable_temporal_fault=0  t_fault=1 s  enable_behavioral_fault=0  max_permissible_current=1 A  t_fail_on_current=1 s  noise_mode=0  sample_time=0.001 s  repeatability=1  auto_seed=178667859  user_seed=0  Tdevice=25 degC  alpha=0.00393 1/K  Tmeas=25 degC  thermal_mass=100 J/K  initial_temperature=25 degC  power_derating_T1=70 degC  power_derating_T2=155 degC  operating_temperature_range_vec=[ -50 150 ] degC
  R2 : elec_lib/Passive Devices/Resistor  R=100e3 Ohm  R_tol=5  enable_R_tol=0  tol_distribution=1  nSigma=4  enable_operating_limits=0  operating_limit_action=2  max_working_voltage=100 V  power_rating=1 W  enable_faults=0  fault_action=1  R_faulted=Inf Ohm  enable_temporal_fault=0  t_fault=1 s  enable_behavioral_fault=0  max_permissible_current=1 A  t_fail_on_current=1 s  noise_mode=0  sample_time=0.001 s  repeatability=1  auto_seed=3261083418  user_seed=0  Tdevice=25 degC  alpha=0.00393 1/K  Tmeas=25 degC  thermal_mass=100 J/K  initial_temperature=25 degC  power_derating_T1=70 degC  power_derating_T2=155 degC  operating_temperature_range_vec=[ -50 150 ] degC
  R3 : elec_lib/Passive Devices/Resistor  R=100e3 Ohm  R_tol=5  enable_R_tol=0  tol_distribution=1  nSigma=4  enable_operating_limits=0  operating_limit_action=2  max_working_voltage=100 V  power_rating=1 W  enable_faults=0  fault_action=1  R_faulted=Inf Ohm  enable_temporal_fault=0  t_fault=1 s  enable_behavioral_fault=0  max_permissible_current=1 A  t_fail_on_current=1 s  noise_mode=0  sample_time=0.001 s  repeatability=1  auto_seed=1395325325  user_seed=0  Tdevice=25 degC  alpha=0.00393 1/K  Tmeas=25 degC  thermal_mass=100 J/K  initial_temperature=25 degC  power_derating_T1=70 degC  power_derating_T2=155 degC  operating_temperature_range_vec=[ -50 150 ] degC
  R4 : elec_lib/Passive Devices/Resistor  R=220e3 Ohm  R_tol=5  enable_R_tol=0  tol_distribution=1  nSigma=4  enable_operating_limits=0  operating_limit_action=2  max_working_voltage=100 V  power_rating=1 W  enable_faults=0  fault_action=1  R_faulted=Inf Ohm  enable_temporal_fault=0  t_fault=1 s  enable_behavioral_fault=0  max_permissible_current=1 A  t_fail_on_current=1 s  noise_mode=0  sample_time=0.001 s  repeatability=1  auto_seed=2241207619  user_seed=0  Tdevice=25 degC  alpha=0.00393 1/K  Tmeas=25 degC  thermal_mass=100 J/K  initial_temperature=25 degC  power_derating_T1=70 degC  power_derating_T2=155 degC  operating_temperature_range_vec=[ -50 150 ] degC
  R5 : elec_lib/Passive Devices/Resistor  R=22e3 Ohm  R_tol=5  enable_R_tol=0  tol_distribution=1  nSigma=4  enable_operating_limits=0  operating_limit_action=2  max_working_voltage=100 V  power_rating=1 W  enable_faults=0  fault_action=1  R_faulted=Inf Ohm  enable_temporal_fault=0  t_fault=1 s  enable_behavioral_fault=0  max_permissible_current=1 A  t_fail_on_current=1 s  noise_mode=0  sample_time=0.001 s  repeatability=1  auto_seed=4088327323  user_seed=0  Tdevice=25 degC  alpha=0.00393 1/K  Tmeas=25 degC  thermal_mass=100 J/K  initial_temperature=25 degC  power_derating_T1=70 degC  power_derating_T2=155 degC  operating_temperature_range_vec=[ -50 150 ] degC
  R6 : elec_lib/Passive Devices/Resistor  R=47e3 Ohm  R_tol=5  enable_R_tol=0  tol_distribution=1  nSigma=4  enable_operating_limits=0  operating_limit_action=2  max_working_voltage=100 V  power_rating=1 W  enable_faults=0  fault_action=1  R_faulted=Inf Ohm  enable_temporal_fault=0  t_fault=1 s  enable_behavioral_fault=0  max_permissible_current=1 A  t_fail_on_current=1 s  noise_mode=0  sample_time=0.001 s  repeatability=1  auto_seed=2873240422  user_seed=0  Tdevice=25 degC  alpha=0.00393 1/K  Tmeas=25 degC  thermal_mass=100 J/K  initial_temperature=25 degC  power_derating_T1=70 degC  power_derating_T2=155 degC  operating_temperature_range_vec=[ -50 150 ] degC
  R7 : elec_lib/Passive Devices/Resistor  R=100e3 Ohm  R_tol=5  enable_R_tol=0  tol_distribution=1  nSigma=4  enable_operating_limits=0  operating_limit_action=2  max_working_voltage=100 V  power_rating=1 W  enable_faults=0  fault_action=1  R_faulted=Inf Ohm  enable_temporal_fault=0  t_fault=1 s  enable_behavioral_fault=0  max_permissible_current=1 A  t_fail_on_current=1 s  noise_mode=0  sample_time=0.001 s  repeatability=1  auto_seed=2032041889  user_seed=0  Tdevice=25 degC  alpha=0.00393 1/K  Tmeas=25 degC  thermal_mass=100 J/K  initial_temperature=25 degC  power_derating_T1=70 degC  power_derating_T2=155 degC  operating_temperature_range_vec=[ -50 150 ] degC
  VDD : PMIOPort  Port=1  Side=Left
  GND : PMIOPort  Port=2  Side=Left
  VSS : PMIOPort  Port=3  Side=Left
  +Vel : PMIOPort  Port=4  Side=Right
  -Vel : PMIOPort  Port=5  Side=Right
  connections:
  P5/LConn1 -- P5/RConn3 -- R4/LConn1 -- P4/LConn1
  R6/LConn1 -- P5/RConn2 -- P5/RConn1 -- N6/RConn3 -- R1/LConn1 -- P1/RConn1 -- P1/RConn2 -- P2/RConn2 -- P2/RConn1 -- P3/RConn1 -- P3/RConn2 -- P4/RConn1 -- P4/RConn2 -- VDD/RConn1
  N2/LConn1 -- R7/RConn1 -- R5/RConn1 -- GND/RConn1 -- R4/RConn1
  N6/RConn2 -- N4/RConn1 -- N4/RConn2 -- N1/RConn2 -- N3/RConn1 -- N3/RConn2 -- N2/RConn2 -- N5/RConn1 -- N5/RConn2 -- VSS/RConn1
  N6/RConn1 -- R7/LConn1 -- R2/LConn1 -- +Vel/RConn1
  R5/LConn1 -- C1/RConn1 -- R6/RConn1
  P4/RConn3 -- N6/LConn1 -- C1/LConn1
  R3/RConn1 -- P3/RConn3 -- -Vel/RConn1 -- N5/RConn3
  N3/LConn1 -- N5/LConn1 -- N4/RConn3 -- R1/RConn1 -- N4/LConn1
  R3/LConn1 -- R2/RConn1 -- N1/LConn1
  P3/LConn1 -- P2/RConn3 -- N2/RConn3
  N3/RConn3 -- N1/RConn1 -- N2/RConn1
  P1/RConn3 -- P1/LConn1 -- P2/LConn1 -- N1/RConn3

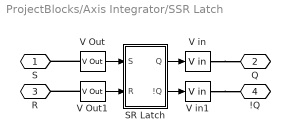
== system ProjectBlocks/Axis Integrator/SSR Latch ==
  SR Latch : Subsystem
  V Out : SimscapeMacros/V Out
  V Out1 : SimscapeMacros/V Out
  V in : SimscapeMacros/V in
  V in1 : SimscapeMacros/V in
  S : PMIOPort  Port=1  Side=Left
  Q : PMIOPort  Port=2  Side=Right
  R : PMIOPort  Port=3  Side=Left
  !Q : PMIOPort  Port=4  Side=Right
  wires:
  SR Latch/1(Q) -> V in/1
  V Out1/1 -> SR Latch/2(R)
  SR Latch/2(!Q) -> V in1/1
  V Out/1 -> SR Latch/1(S)
  connections:
  V in/RConn1 -- Q/RConn1
  V Out/LConn1 -- S/RConn1
  V in1/RConn1 -- !Q/RConn1
  V Out1/LConn1 -- R/RConn1

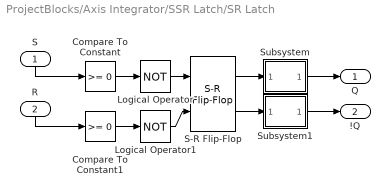
== system ProjectBlocks/Axis Integrator/SSR Latch/SR Latch ==
  S : Inport
  R : Inport  Port=2
  Compare To Constant : simulink/Logic and Bit Operations/Compare To Constant  relop=>=  const=0  OutDataTypeStr=boolean
  Compare To Constant1 : simulink/Logic and Bit Operations/Compare To Constant  relop=>=  const=0  OutDataTypeStr=boolean
  Logical Operator : Logic  Operator=NOT  AllPortsSameDT=off  OutDataTypeStr=boolean
  Logical Operator1 : Logic  Operator=NOT  AllPortsSameDT=off  OutDataTypeStr=boolean
  S-R Flip-Flop : simulink_extras/Flip Flops/S-R Flip-Flop  initial_condition=1
  Subsystem : Subsystem
  Subsystem1 : Subsystem
  Q : Outport
  !Q : Outport  Port=2
  wires:
  Logical Operator1/1 -> S-R Flip-Flop/2
  Logical Operator/1 -> S-R Flip-Flop/1
  S/1 -> Compare To Constant/1
  R/1 -> Compare To Constant1/1
  Compare To Constant1/1 -> Logical Operator1/1
  S-R Flip-Flop/2 -> Subsystem1/1(In1)
  Compare To Constant/1 -> Logical Operator/1
  Subsystem1/1(Out1) -> !Q/1
  Subsystem/1(Out1) -> Q/1
  S-R Flip-Flop/1 -> Subsystem/1(In1)

== system ProjectBlocks/Axis Integrator/SSR Latch/SR Latch/Subsystem ==
  In1 : Inport
  Constant1 : Constant  Value=10
  Gain : Gain  Gain=20
  Subtract1 : Sum  Inputs=+-
  Out1 : Outport
  wires:
  Gain/1 -> Subtract1/1
  Constant1/1 -> Subtract1/2
  In1/1 -> Gain/1
  Subtract1/1 -> Out1/1

== system ProjectBlocks/Axis Integrator/SSR Latch/SR Latch/Subsystem1 ==
  In1 : Inport
  Constant1 : Constant  Value=10
  Gain : Gain  Gain=20
  Subtract1 : Sum  Inputs=+-
  Out1 : Outport
  wires:
  Gain/1 -> Subtract1/1
  Constant1/1 -> Subtract1/2
  In1/1 -> Gain/1
  Subtract1/1 -> Out1/1
